simulink library "Powertrain_Library_GenAI"  (R2024a)
settings: Solver=VariableStepAuto  StartTime=0.0  StopTime=10.0  RelTol=1e-3
undefined symbols (not defined in the file or in its folder): DriveCycle
libraries: simulink x8, slpidlib x1
(part 2 of 2)

== system Powertrain_Library_GenAI/IC Engine/ICE_Torque_Limits ==
  T_req : Inport
  w_ice : Inport  Port=2
  Normalized 3rd-order polynomial based : Subsystem  VariantControl=Normalized 3rd-order polynomial approximation
  Torque curve data based : Subsystem  VariantControl=Torque-Speed curve data
  T_ice : Outport
  w_ice_p : Outport  Port=2
  T_ice_norm : Outport  Port=3
  w_ice_pnorm : Outport  Port=4

== system Powertrain_Library_GenAI/Motor/Mot_Efficiency ==
  T_mot_norm : Inport
  w_mot_norm : Inport  Port=2
  Constant Efficiency : Subsystem  VariantControl=Constant Efficiency
  Variable Efficiency : Subsystem  VariantControl=Variable Efficiency
  eff_mot : Outport

== system Powertrain_Library_GenAI/IC Engine/ICE_Efficiency/Average Efficiency ==
  Constant1 : Constant  Value=eff_ice_avg
  eff_ice : Outport
  wires:
  Constant1/1 -> eff_ice/1

== system Powertrain_Library_GenAI/IC Engine/ICE_Efficiency/Efficiency Map ==
  T_ice_norm : Inport
  w_ice_pnorm : Inport  Port=2
  2-D Lookup Table : Lookup_n-D  BreakpointsForDimension1=T_ice_norm_data  BreakpointsForDimension2=w_ice_norm_data  Table=eff_ice_data  InternalRulePriority=Speed  RndMeth=Simplest
      settings: InputPortMap=u0,u1
  eff_ice : Outport
  wires:
  2-D Lookup Table/1 -> eff_ice/1  "eff_ice"
  w_ice_pnorm/1 -> 2-D Lookup Table/2
  T_ice_norm/1 -> 2-D Lookup Table/1

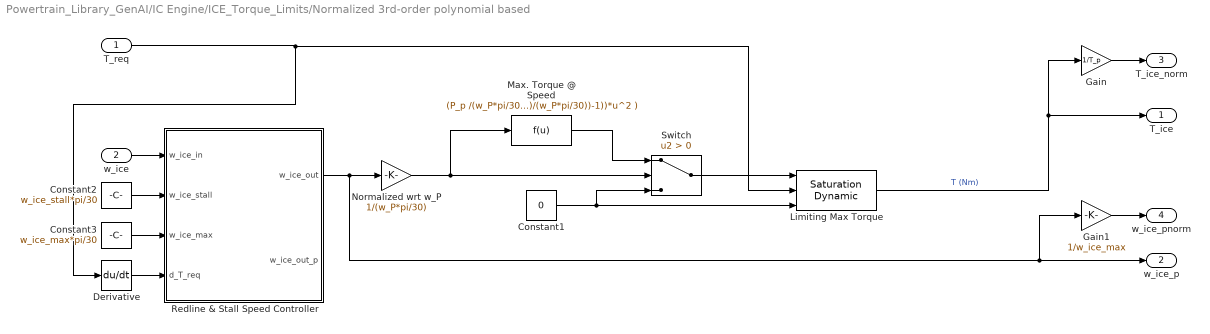
== system Powertrain_Library_GenAI/IC Engine/ICE_Torque_Limits/Normalized 3rd-order polynomial based ==
  T_req : Inport
  w_ice : Inport  Port=2
  Constant1 : Constant  Value=0
  Constant2 : Constant  Value=w_ice_stall*pi/30
  Constant3 : Constant  Value=w_ice_max*pi/30
  Derivative : Derivative
  Gain : Gain  Gain=1/T_p
  Gain1 : Gain  Gain=1/w_ice_max
  Limiting Max Torque : simulink/Discontinuities/Saturation Dynamic  OutMin=[]  OutMax=[]  OutDataTypeStr=Inherit: Same as second input  OutDataType=fixdt(1, 16)  OutScaling=2^-10  DoSatur=off
  Max. Torque @ Speed : Fcn  Expr=(P_p /(w_P*pi/30)) *( ((3-4*((w_T*pi/30)/(w_P*pi/30)))/(2*(1-((w_T*pi/30)/(w_P*pi/30))))) + (-((w_T*pi/30)/(w_P*pi/30))/(((w_T*pi/30)/(w_P*pi/30))-1))*u + (0.5/(((w_T*pi/30)/(w_P*pi/30))-1))*u^2 )
  Normalized wrt w_P : Gain  Gain=1/(w_P*pi/30)
  Redline & Stall Speed Controller : MATLAB Function  TreatAsAtomicUnit=on
  Switch : Switch  Criteria=u2 > Threshold  SaturateOnIntegerOverflow=off  InputSameDT=off
  T_ice : Outport
  w_ice_p : Outport  Port=2
  T_ice_norm : Outport  Port=3
  w_ice_pnorm : Outport  Port=4
  wires:
  Normalized wrt w_P/1 -> Max. Torque @ Speed/1, Switch/2
  Constant3/1 -> Redline & Stall Speed Controller/3(w_ice_max)
  Constant2/1 -> Redline & Stall Speed Controller/2(w_ice_stall)
  Derivative/1 -> Redline & Stall Speed Controller/4(d_T_req)
  T_req/1 -> Derivative/1, Limiting Max Torque/2
  Gain/1 -> T_ice_norm/1
  Limiting Max Torque/1 -> Gain/1, T_ice/1  "T (Nm)"
  Gain1/1 -> w_ice_pnorm/1
  Redline & Stall Speed Controller/1(w_ice_out) -> Gain1/1, w_ice_p/1, Normalized wrt w_P/1
  Max. Torque @ Speed/1 -> Switch/1
  Constant1/1 -> Limiting Max Torque/3, Switch/3
  Switch/1 -> Limiting Max Torque/1
  w_ice/1 -> Redline & Stall Speed Controller/1(w_ice_in)

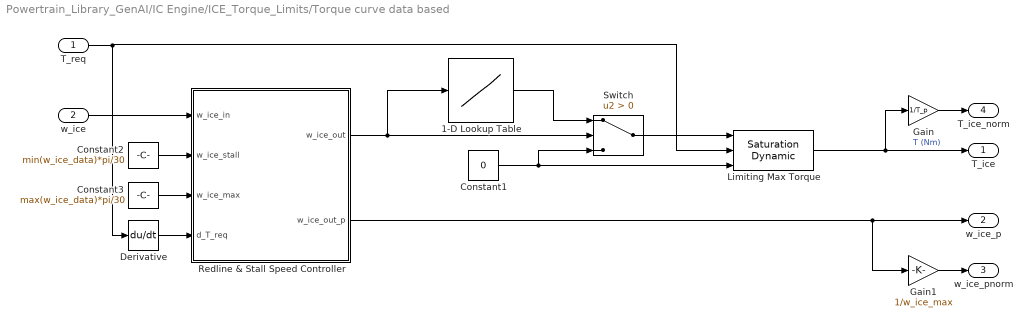
== system Powertrain_Library_GenAI/IC Engine/ICE_Torque_Limits/Torque curve data based ==
  T_req : Inport
  w_ice : Inport  Port=2
  1-D Lookup Table : Lookup_n-D  NumberOfTableDimensions=1  BreakpointsForDimension1=w_ice_data  Table=T_ice_data  InternalRulePriority=Speed  RndMeth=Simplest
  Constant1 : Constant  Value=0
  Constant2 : Constant  Value=min(w_ice_data)*pi/30
  Constant3 : Constant  Value=max(w_ice_data)*pi/30
  Derivative : Derivative
  Gain : Gain  Gain=1/T_p
  Gain1 : Gain  Gain=1/w_ice_max
  Limiting Max Torque : simulink/Discontinuities/Saturation Dynamic  OutMin=[]  OutMax=[]  OutDataTypeStr=Inherit: Same as second input  OutDataType=fixdt(1, 16)  OutScaling=2^-10  DoSatur=off
  Redline & Stall Speed Controller : MATLAB Function  TreatAsAtomicUnit=on
  Switch : Switch  Criteria=u2 > Threshold  SaturateOnIntegerOverflow=off  InputSameDT=off
  T_ice : Outport
  w_ice_p : Outport  Port=2
  w_ice_pnorm : Outport  Port=3
  T_ice_norm : Outport  Port=4
  wires:
  Limiting Max Torque/1 -> T_ice/1, Gain/1  "T (Nm)"
  Redline & Stall Speed Controller/1(w_ice_out) -> 1-D Lookup Table/1, Switch/2
  w_ice/1 -> Redline & Stall Speed Controller/1(w_ice_in)
  Constant2/1 -> Redline & Stall Speed Controller/2(w_ice_stall)
  Derivative/1 -> Redline & Stall Speed Controller/4(d_T_req)
  Constant3/1 -> Redline & Stall Speed Controller/3(w_ice_max)
  T_req/1 -> Limiting Max Torque/2, Derivative/1
  Gain1/1 -> w_ice_pnorm/1
  Gain/1 -> T_ice_norm/1
  1-D Lookup Table/1 -> Switch/1
  Switch/1 -> Limiting Max Torque/1
  Constant1/1 -> Limiting Max Torque/3, Switch/3
  Redline & Stall Speed Controller/2(w_ice_out_p) -> Gain1/1, w_ice_p/1

== system Powertrain_Library_GenAI/Motor/Mot_Efficiency/Constant Efficiency ==
  Constant : Constant  Value=eff_mot_avg
  eff_mot : Outport
  wires:
  Constant/1 -> eff_mot/1

== system Powertrain_Library_GenAI/Motor/Mot_Efficiency/Variable Efficiency ==
  T_mot_norm : Inport
  w_mot_norm : Inport  Port=2
  2-D Lookup Table : Lookup_n-D  LookupTableObject=''  BreakpointsSpecification=Even spacing  BreakpointsForDimension1=T_mot_norm_data  BreakpointsForDimension2=w_mot_norm_data  BreakpointsForDimension1FirstPoint=0  BreakpointsForDimension2FirstPoint=0  BreakpointsForDimension1Spacing=0.025  BreakpointsForDimension2Spacing=0.0312  BreakpointsForDimension1DataTypeStr=double  BreakpointsForDimension2DataTypeStr=double  IndexSearchMethod=Evenly spaced points  Table=eff_mot_data  TableDataTypeStr=double  InterpMethod=Flat  DiagnosticForOutOfRangeInput=Error  OutDataTypeStr=double  RndMeth=Simplest
      settings: InputPortMap=u0,u1
  eff_mot : Outport
  wires:
  T_mot_norm/1 -> 2-D Lookup Table/1
  w_mot_norm/1 -> 2-D Lookup Table/2
  2-D Lookup Table/1 -> eff_mot/1

== matlab function Powertrain_Library_GenAI/Driver/MATLAB Function ==
  data: SOC input; signal output; time input; min_charge_SOC input; charging_time input; charging_torque input; off_time_in input; off_time_out output
function [signal, off_time_out] = fcn(SOC, time, min_charge_SOC, charging_time, charging_torque, off_time_in)
    if SOC >= 1 % If the battery is fully charged
        signal = 0; % Turn off the engine, regardless of other conditions
        off_time_out = off_time_in;
    elseif SOC <= min_charge_SOC % If SOC is less than minimum allowed (engine needed)
        signal = charging_torque;            % Turn on the engine
        off_time_out = time + charging_time; % Set the stop time
    elseif time <= off_time_in % If SOC is more than minimum allowed (engine not needed) but stop time not yet 
        signal = charging_torque;   % Keep the engine on
        off_time_out = off_time_in; % Keep the same stop time
    else % If SOC is more than minimum allowed (engine not needed), stop time is here
        signal = 0; % Turn the engine off
        off_time_out = off_time_in; % Keep the same stop time (doesnt matter, will be updated once engine is on again)
    end
end

== matlab function Powertrain_Library_GenAI/Transmission/MATLAB Function ==
  data: v input; gear output; Gs input; shift_thresholds input
function gear = fcn(v, Gs, shift_thresholds)
for i = 1:numel(shift_thresholds)
    if v <= shift_thresholds(i)
        gear = Gs(i);
        break;
    elseif v > shift_thresholds(length(shift_thresholds))
        gear = Gs(length(Gs));
    else
        gear = Gs(1);
    end 
end

== matlab function Powertrain_Library_GenAI/IC Engine/ICE_Torque_Limits/Normalized 3rd-order polynomial based/Redline & Stall Speed Controller ==
  data: w_ice_in input; w_ice_out output; w_ice_stall input; w_ice_max input; d_T_req input; w_ice_out_p output
function [w_ice_out, w_ice_out_p] = fcn(w_ice_in, w_ice_stall, w_ice_max, d_T_req)

if w_ice_in < w_ice_stall
    w_ice_out_p = w_ice_stall;
    if d_T_req < 0
        w_ice_out = 0;
    else 
        w_ice_out = w_ice_stall;
        %w_ice_out = 0;
    end 
elseif w_ice_in > w_ice_max
    w_ice_out = 0;
    w_ice_out_p = w_ice_max;
else 
    w_ice_out = w_ice_in;
    w_ice_out_p = w_ice_in;
end

== matlab function Powertrain_Library_GenAI/IC Engine/ICE_Torque_Limits/Torque curve data based/Redline & Stall Speed Controller ==
  data: w_ice_in input; w_ice_out output; w_ice_stall input; w_ice_max input; d_T_req input; w_ice_out_p output
function [w_ice_out, w_ice_out_p] = fcn(w_ice_in, w_ice_stall, w_ice_max, d_T_req)

if w_ice_in < w_ice_stall
    w_ice_out_p = w_ice_stall;
    if d_T_req < 0
        w_ice_out = 0;
    else 
        w_ice_out = w_ice_stall;
    end 
elseif w_ice_in > w_ice_max
    w_ice_out = 0;
    w_ice_out_p = w_ice_max;
else 
    w_ice_out = w_ice_in;
    w_ice_out_p = w_ice_in;
end
